simulink model "MSBR_Plant"  (R2021b)
settings: Solver=ode45  StartTime=0.0  StopTime=sim_time  MaxStep=ts_max  RelTol=1e-4
values from neighbouring files (symbols this model uses):
  a_1 = 8.7292e-2/wilson_ratio    (= 0.0087292)    [Whole_Plant_Cool_Pump_Accident_script.m]    (also in Whole_Plant_Fert_Pump_Accident_script.m; Whole_Plant_Fuel_Pump_Accident.m; Whole_Plant_Fuel_Pump_Accident_script.m; Whole_Plant_Reactivity_Accident.m)
  a_2 = 7.3787e-4/wilson_ratio    (= 7.3787e-05)    [Whole_Plant_Cool_Pump_Accident_script.m]    (also in Whole_Plant_Fert_Pump_Accident_script.m; Whole_Plant_Fuel_Pump_Accident.m; Whole_Plant_Fuel_Pump_Accident_script.m; Whole_Plant_Reactivity_Accident.m)
  a_b = 1.656e-5    (= 1.656e-05)    [Whole_Plant_Cool_Pump_Accident_script.m]    (also in Whole_Plant_Fert_Pump_Accident_script.m; Whole_Plant_Fuel_Pump_Accident.m; Whole_Plant_Fuel_Pump_Accident_script.m; Whole_Plant_Reactivity_Accident.m)
  a_f = -8.172e-5    (= -8.172e-05)    [Whole_Plant_Cool_Pump_Accident_script.m]    (also in Whole_Plant_Fert_Pump_Accident_script.m; Whole_Plant_Fuel_Pump_Accident.m; Whole_Plant_Fuel_Pump_Accident_script.m; Whole_Plant_Reactivity_Accident.m)
  a_g = 2.016e-5    (= 2.016e-05)    [Whole_Plant_Cool_Pump_Accident_script.m]    (also in Whole_Plant_Fert_Pump_Accident_script.m; Whole_Plant_Fuel_Pump_Accident.m; Whole_Plant_Fuel_Pump_Accident_script.m; Whole_Plant_Reactivity_Accident.m)
  A_s = pi()*((D_OTSG_i^2)/4) - A_w_OTSG - A_p_OTSG    [Whole_Plant_Cool_Pump_Accident_script.m]    (also in Whole_Plant_Fert_Pump_Accident_script.m; Whole_Plant_Fuel_Pump_Accident.m; Whole_Plant_Fuel_Pump_Accident_script.m; Whole_Plant_Reactivity_Accident.m)
  alpha_co = 316.2    [Whole_Plant_Cool_Pump_Accident_script.m]    (also in Whole_Plant_Fert_Pump_Accident_script.m; Whole_Plant_Fuel_Pump_Accident.m; Whole_Plant_Fuel_Pump_Accident_script.m; Whole_Plant_Reactivity_Accident.m)
  beta = [2.290e-04, 8.320e-04, 7.100e-04, 8.520e-04, 1.710e-04, 1.020e-04]    [Whole_Plant_Cool_Pump_Accident_script.m]    (also in Whole_Plant_Fert_Pump_Accident_script.m; Whole_Plant_Fuel_Pump_Accident.m; Whole_Plant_Fuel_Pump_Accident_script.m; Whole_Plant_Reactivity_Accident.m)
  beta_co = 68.0958    [Whole_Plant_Cool_Pump_Accident_script.m]    (also in Whole_Plant_Fert_Pump_Accident_script.m; Whole_Plant_Fuel_Pump_Accident.m; Whole_Plant_Fuel_Pump_Accident_script.m; Whole_Plant_Reactivity_Accident.m)
  beta_t = sum(beta)    [Whole_Plant_Cool_Pump_Accident_script.m]    (also in Whole_Plant_Fert_Pump_Accident_script.m; Whole_Plant_Fuel_Pump_Accident.m; Whole_Plant_Fuel_Pump_Accident_script.m; Whole_Plant_Reactivity_Accident.m)
  C_nc_X_A_nc = 12.8    [Whole_Plant_Cool_Pump_Accident_script.m]    (also in Whole_Plant_Fert_Pump_Accident_script.m; Whole_Plant_Fuel_Pump_Accident.m; Whole_Plant_Fuel_Pump_Accident_script.m; Whole_Plant_Reactivity_Accident.m)
  C_pcw = 0.0042    [Whole_Plant_Cool_Pump_Accident_script.m]    (also in Whole_Plant_Fert_Pump_Accident_script.m; Whole_Plant_Fuel_Pump_Accident.m; Whole_Plant_Fuel_Pump_Accident_script.m; Whole_Plant_Reactivity_Accident.m)
  C_rh_X_A_rh = 33    [Whole_Plant_Cool_Pump_Accident_script.m]    (also in Whole_Plant_Fert_Pump_Accident_script.m; Whole_Plant_Fuel_Pump_Accident.m; Whole_Plant_Fuel_Pump_Accident_script.m; Whole_Plant_Reactivity_Accident.m)
  C_v = 0.84    [Whole_Plant_Cool_Pump_Accident_script.m]    (also in Whole_Plant_Fert_Pump_Accident_script.m; Whole_Plant_Fuel_Pump_Accident.m; Whole_Plant_Fuel_Pump_Accident_script.m; Whole_Plant_Reactivity_Accident.m)
  ce1 = 1.2471e-07    [Whole_Plant_Cool_Pump_Accident_script.m]    (also in Whole_Plant_Fert_Pump_Accident_script.m; Whole_Plant_Fuel_Pump_Accident.m; Whole_Plant_Fuel_Pump_Accident_script.m; Whole_Plant_Reactivity_Accident.m)
  ce2 = 5.3816e-14    [Whole_Plant_Cool_Pump_Accident_script.m]    (also in Whole_Plant_Fert_Pump_Accident_script.m; Whole_Plant_Fuel_Pump_Accident.m; Whole_Plant_Fuel_Pump_Accident_script.m; Whole_Plant_Reactivity_Accident.m)
  ce3 = 3.3721e-08    [Whole_Plant_Cool_Pump_Accident_script.m]    (also in Whole_Plant_Fert_Pump_Accident_script.m; Whole_Plant_Fuel_Pump_Accident.m; Whole_Plant_Fuel_Pump_Accident_script.m; Whole_Plant_Reactivity_Accident.m)
  Cp_fw = XSteam('Cp_pT',P_set*10,T_fw)/1000    [Whole_Plant_Cool_Pump_Accident_script.m]    (also in Whole_Plant_Fert_Pump_Accident_script.m; Whole_Plant_Fuel_Pump_Accident.m; Whole_Plant_Fuel_Pump_Accident_script.m; Whole_Plant_Reactivity_Accident.m)
  Cp_p = Cp_sec    (= 0.001716588)    [Whole_Plant_Cool_Pump_Accident_script.m]    (also in Whole_Plant_Fert_Pump_Accident_script.m; Whole_Plant_Fuel_Pump_Accident.m; Whole_Plant_Fuel_Pump_Accident_script.m; Whole_Plant_Reactivity_Accident.m)
  Cp_rh = 0.0021520    (= 0.002152)    [Whole_Plant_Cool_Pump_Accident_script.m]    (also in Whole_Plant_Fert_Pump_Accident_script.m; Whole_Plant_Fuel_Pump_Accident.m; Whole_Plant_Fuel_Pump_Accident_script.m; Whole_Plant_Reactivity_Accident.m)
  Cp_s = XSteam('Cp_pT',P_s*10,T_s)/1000    [Whole_Plant_Cool_Pump_Accident_script.m]    (also in Whole_Plant_Fert_Pump_Accident_script.m; Whole_Plant_Fuel_Pump_Accident.m; Whole_Plant_Fuel_Pump_Accident_script.m; Whole_Plant_Reactivity_Accident.m)
  Cp_sc = XSteam('Cp_pT',P_set*10,T_sc2)/1000    [Whole_Plant_Cool_Pump_Accident_script.m]    (also in Whole_Plant_Fert_Pump_Accident_script.m; Whole_Plant_Fuel_Pump_Accident.m; Whole_Plant_Fuel_Pump_Accident_script.m; Whole_Plant_Reactivity_Accident.m)
  Cp_w = 468.992e-6    (= 0.000468992)    [Whole_Plant_Cool_Pump_Accident_script.m]    (also in Whole_Plant_Fert_Pump_Accident_script.m; Whole_Plant_Fuel_Pump_Accident.m; Whole_Plant_Fuel_Pump_Accident_script.m; Whole_Plant_Reactivity_Accident.m)
  D_it = D_ot-2*T_th    (= 0.014147)    [Whole_Plant_Cool_Pump_Accident_script.m]    (also in Whole_Plant_Fert_Pump_Accident_script.m; Whole_Plant_Fuel_Pump_Accident.m; Whole_Plant_Fuel_Pump_Accident_script.m; Whole_Plant_Reactivity_Accident.m)
  D_ot = 0.015875    [Whole_Plant_Cool_Pump_Accident_script.m]    (also in Whole_Plant_Fert_Pump_Accident_script.m; Whole_Plant_Fuel_Pump_Accident.m; Whole_Plant_Fuel_Pump_Accident_script.m; Whole_Plant_Reactivity_Accident.m)
  dHs_dPs = c(1)    [Whole_Plant_Cool_Pump_Accident_script.m]    (also in Whole_Plant_Fert_Pump_Accident_script.m; Whole_Plant_Fuel_Pump_Accident.m; Whole_Plant_Fuel_Pump_Accident_script.m; Whole_Plant_Reactivity_Accident.m)
  eta_hp_isen = 0.861    [Whole_Plant_Cool_Pump_Accident_script.m]    (also in Whole_Plant_Fert_Pump_Accident_script.m; Whole_Plant_Fuel_Pump_Accident.m; Whole_Plant_Fuel_Pump_Accident_script.m; Whole_Plant_Reactivity_Accident.m)
  eta_lp_isen = 0.861    [Whole_Plant_Cool_Pump_Accident_script.m]    (also in Whole_Plant_Fert_Pump_Accident_script.m; Whole_Plant_Fuel_Pump_Accident.m; Whole_Plant_Fuel_Pump_Accident_script.m; Whole_Plant_Reactivity_Accident.m)
  gamma_I = 5.1135e-2    (= 0.051135)    [Whole_Plant_Cool_Pump_Accident_script.m]    (also in Whole_Plant_Fert_Pump_Accident_script.m; Whole_Plant_Fuel_Pump_Accident.m; Whole_Plant_Fuel_Pump_Accident_script.m; Whole_Plant_Reactivity_Accident.m)
  gamma_Xe = 1.1628e-2    (= 0.011628)    [Whole_Plant_Cool_Pump_Accident_script.m]    (also in Whole_Plant_Fert_Pump_Accident_script.m; Whole_Plant_Fuel_Pump_Accident.m; Whole_Plant_Fuel_Pump_Accident_script.m; Whole_Plant_Reactivity_Accident.m)
  H_co0 = 0.149    [Whole_Plant_Cool_Pump_Accident_script.m]    (also in Whole_Plant_Fert_Pump_Accident_script.m; Whole_Plant_Fuel_Pump_Accident.m; Whole_Plant_Fuel_Pump_Accident_script.m; Whole_Plant_Reactivity_Accident.m)
  H_f_co0 = 0.149    [Whole_Plant_Cool_Pump_Accident_script.m]    (also in Whole_Plant_Fert_Pump_Accident_script.m; Whole_Plant_Fuel_Pump_Accident.m; Whole_Plant_Fuel_Pump_Accident_script.m; Whole_Plant_Reactivity_Accident.m)
  H_fg_co0 = 2.35    [Whole_Plant_Cool_Pump_Accident_script.m]    (also in Whole_Plant_Fert_Pump_Accident_script.m; Whole_Plant_Fuel_Pump_Accident.m; Whole_Plant_Fuel_Pump_Accident_script.m; Whole_Plant_Reactivity_Accident.m)
  H_fgrh0 = (XSteam('hV_p', P_s*1e1) - XSteam('hL_p', P_s*1e1))/1e3    [Whole_Plant_Cool_Pump_Accident_script.m]    (also in Whole_Plant_Fert_Pump_Accident_script.m; Whole_Plant_Fuel_Pump_Accident.m; Whole_Plant_Fuel_Pump_Accident_script.m; Whole_Plant_Reactivity_Accident.m)
  H_frh0 = XSteam('hL_p', P_s*1e1)/1e3    [Whole_Plant_Cool_Pump_Accident_script.m]    (also in Whole_Plant_Fert_Pump_Accident_script.m; Whole_Plant_Fuel_Pump_Accident.m; Whole_Plant_Fuel_Pump_Accident_script.m; Whole_Plant_Reactivity_Accident.m)
  h_fwh1 = 0.5927    [Whole_Plant_Cool_Pump_Accident_script.m]    (also in Whole_Plant_Fert_Pump_Accident_script.m; Whole_Plant_Fuel_Pump_Accident.m; Whole_Plant_Fuel_Pump_Accident_script.m; Whole_Plant_Reactivity_Accident.m)
  H_fwh10 = 0.46009    [Whole_Plant_Cool_Pump_Accident_script.m]    (also in Whole_Plant_Fert_Pump_Accident_script.m; Whole_Plant_Fuel_Pump_Accident.m; Whole_Plant_Fuel_Pump_Accident_script.m; Whole_Plant_Reactivity_Accident.m)
  h_fwh2 = 1.230803    [Whole_Plant_Cool_Pump_Accident_script.m]    (also in Whole_Plant_Fert_Pump_Accident_script.m; Whole_Plant_Fuel_Pump_Accident.m; Whole_Plant_Fuel_Pump_Accident_script.m; Whole_Plant_Reactivity_Accident.m)
  H_fwh20 = 0.6784    [Whole_Plant_Cool_Pump_Accident_script.m]    (also in Whole_Plant_Fert_Pump_Accident_script.m; Whole_Plant_Fuel_Pump_Accident.m; Whole_Plant_Fuel_Pump_Accident_script.m; Whole_Plant_Reactivity_Accident.m)
  H_grh0 = 2.8029    [Whole_Plant_Cool_Pump_Accident_script.m]    (also in Whole_Plant_Fert_Pump_Accident_script.m; Whole_Plant_Fuel_Pump_Accident.m; Whole_Plant_Fuel_Pump_Accident_script.m; Whole_Plant_Reactivity_Accident.m)
  H_hp_isen0 = 2.5111    [Whole_Plant_Cool_Pump_Accident_script.m]    (also in Whole_Plant_Fert_Pump_Accident_script.m; Whole_Plant_Fuel_Pump_Accident.m; Whole_Plant_Fuel_Pump_Accident_script.m; Whole_Plant_Reactivity_Accident.m)
  H_hpt_out = 2.6201    [Whole_Plant_Cool_Pump_Accident_script.m]    (also in Whole_Plant_Fert_Pump_Accident_script.m; Whole_Plant_Fuel_Pump_Accident.m; Whole_Plant_Fuel_Pump_Accident_script.m; Whole_Plant_Reactivity_Accident.m)
  H_lp_isen = 958.4*1054.35e-6/0.45359237    (= 2.22774699671)    [Whole_Plant_Cool_Pump_Accident_script.m]    (also in Whole_Plant_Fert_Pump_Accident_script.m; Whole_Plant_Fuel_Pump_Accident.m; Whole_Plant_Fuel_Pump_Accident_script.m; Whole_Plant_Reactivity_Accident.m)
  H_lpt_out = 2.3089    [Whole_Plant_Cool_Pump_Accident_script.m]    (also in Whole_Plant_Fert_Pump_Accident_script.m; Whole_Plant_Fuel_Pump_Accident.m; Whole_Plant_Fuel_Pump_Accident_script.m; Whole_Plant_Reactivity_Accident.m)
  H_nc = XSteam('h_pT', P_s*10, T_s)/1000    [Whole_Plant_Cool_Pump_Accident_script.m]    (also in Whole_Plant_Fert_Pump_Accident_script.m; Whole_Plant_Fuel_Pump_Accident.m; Whole_Plant_Fuel_Pump_Accident_script.m; Whole_Plant_Reactivity_Accident.m)
  h_pw = h_s    (= 0.02555)    [Whole_Plant_Cool_Pump_Accident_script.m]    (also in Whole_Plant_Fert_Pump_Accident_script.m; Whole_Plant_Fuel_Pump_Accident.m; Whole_Plant_Fuel_Pump_Accident_script.m; Whole_Plant_Reactivity_Accident.m)
  H_rh = 2.8115    [Whole_Plant_Cool_Pump_Accident_script.m]    (also in Whole_Plant_Fert_Pump_Accident_script.m; Whole_Plant_Fuel_Pump_Accident.m; Whole_Plant_Fuel_Pump_Accident_script.m; Whole_Plant_Reactivity_Accident.m)
  h_wb = 13349.334646671E-6    (= 0.0133493346467)    [Whole_Plant_Cool_Pump_Accident_script.m]    (also in Whole_Plant_Fert_Pump_Accident_script.m; Whole_Plant_Fuel_Pump_Accident.m; Whole_Plant_Fuel_Pump_Accident_script.m; Whole_Plant_Reactivity_Accident.m)
  h_ws = 5732.378387768E-6    (= 0.00573237838777)    [Whole_Plant_Cool_Pump_Accident_script.m]    (also in Whole_Plant_Fert_Pump_Accident_script.m; Whole_Plant_Fuel_Pump_Accident.m; Whole_Plant_Fuel_Pump_Accident_script.m; Whole_Plant_Reactivity_Accident.m)
  h_wsc = 8385.005556375E-6    (= 0.00838500555638)    [Whole_Plant_Cool_Pump_Accident_script.m]    (also in Whole_Plant_Fert_Pump_Accident_script.m; Whole_Plant_Fuel_Pump_Accident.m; Whole_Plant_Fuel_Pump_Accident_script.m; Whole_Plant_Reactivity_Accident.m)
  hA_bg = A_fert*h_bg    (= 2.76411813627)    [Whole_Plant_Cool_Pump_Accident_script.m]    (also in Whole_Plant_Fert_Pump_Accident_script.m; Whole_Plant_Fuel_Pump_Accident.m; Whole_Plant_Fuel_Pump_Accident_script.m; Whole_Plant_Reactivity_Accident.m)
  hA_co0 = 140    [Whole_Plant_Cool_Pump_Accident_script.m]    (also in Whole_Plant_Fert_Pump_Accident_script.m; Whole_Plant_Fuel_Pump_Accident.m; Whole_Plant_Fuel_Pump_Accident_script.m; Whole_Plant_Reactivity_Accident.m)
  hA_fg_dn = h_fg*A_fuel_down    [Whole_Plant_Cool_Pump_Accident_script.m]    (also in Whole_Plant_Fert_Pump_Accident_script.m; Whole_Plant_Fuel_Pump_Accident.m; Whole_Plant_Fuel_Pump_Accident_script.m; Whole_Plant_Reactivity_Accident.m)
  hA_fg_up = h_fg*A_fuel_up    [Whole_Plant_Cool_Pump_Accident_script.m]    (also in Whole_Plant_Fert_Pump_Accident_script.m; Whole_Plant_Fuel_Pump_Accident.m; Whole_Plant_Fuel_Pump_Accident_script.m; Whole_Plant_Reactivity_Accident.m)
  hA_p_bhx1 = [h_pb*A_pbhx/2,h_pb*A_pbhx/2]    [Whole_Plant_Cool_Pump_Accident_script.m]    (also in Whole_Plant_Fert_Pump_Accident_script.m; Whole_Plant_Fuel_Pump_Accident.m; Whole_Plant_Fuel_Pump_Accident_script.m; Whole_Plant_Reactivity_Accident.m)
  hA_p_bhx2 = hA_p_bhx1    [Whole_Plant_Cool_Pump_Accident_script.m]    (also in Whole_Plant_Fert_Pump_Accident_script.m; Whole_Plant_Fuel_Pump_Accident.m; Whole_Plant_Fuel_Pump_Accident_script.m; Whole_Plant_Reactivity_Accident.m)
  hA_p_bhx3 = hA_p_bhx1    [Whole_Plant_Cool_Pump_Accident_script.m]    (also in Whole_Plant_Fert_Pump_Accident_script.m; Whole_Plant_Fuel_Pump_Accident.m; Whole_Plant_Fuel_Pump_Accident_script.m; Whole_Plant_Reactivity_Accident.m)
  hA_p_bhx4 = hA_p_bhx1    [Whole_Plant_Cool_Pump_Accident_script.m]    (also in Whole_Plant_Fert_Pump_Accident_script.m; Whole_Plant_Fuel_Pump_Accident.m; Whole_Plant_Fuel_Pump_Accident_script.m; Whole_Plant_Reactivity_Accident.m)
  hA_p_fhx1 = [h_p*A_pfhx_dn/2,h_p*A_pfhx_dn/2,h_p*A_pfhx_up/2,h_p*A_pfhx_up/2]    [Whole_Plant_Cool_Pump_Accident_script.m]    (also in Whole_Plant_Fert_Pump_Accident_script.m; Whole_Plant_Fuel_Pump_Accident.m; Whole_Plant_Fuel_Pump_Accident_script.m; Whole_Plant_Reactivity_Accident.m)
  hA_p_fhx2 = hA_p_fhx1    [Whole_Plant_Cool_Pump_Accident_script.m]    (also in Whole_Plant_Fert_Pump_Accident_script.m; Whole_Plant_Fuel_Pump_Accident.m; Whole_Plant_Fuel_Pump_Accident_script.m; Whole_Plant_Reactivity_Accident.m)
  hA_p_fhx3 = hA_p_fhx1    [Whole_Plant_Cool_Pump_Accident_script.m]    (also in Whole_Plant_Fert_Pump_Accident_script.m; Whole_Plant_Fuel_Pump_Accident.m; Whole_Plant_Fuel_Pump_Accident_script.m; Whole_Plant_Reactivity_Accident.m)
  hA_p_fhx4 = hA_p_fhx1    [Whole_Plant_Cool_Pump_Accident_script.m]    (also in Whole_Plant_Fert_Pump_Accident_script.m; Whole_Plant_Fuel_Pump_Accident.m; Whole_Plant_Fuel_Pump_Accident_script.m; Whole_Plant_Reactivity_Accident.m)
  hA_s_bhx1 = [h_sb*A_sbhx/2,h_sb*A_sbhx/2]    [Whole_Plant_Cool_Pump_Accident_script.m]    (also in Whole_Plant_Fert_Pump_Accident_script.m; Whole_Plant_Fuel_Pump_Accident.m; Whole_Plant_Fuel_Pump_Accident_script.m; Whole_Plant_Reactivity_Accident.m)
  hA_s_bhx2 = hA_s_bhx1    [Whole_Plant_Cool_Pump_Accident_script.m]    (also in Whole_Plant_Fert_Pump_Accident_script.m; Whole_Plant_Fuel_Pump_Accident.m; Whole_Plant_Fuel_Pump_Accident_script.m; Whole_Plant_Reactivity_Accident.m)
  hA_s_bhx3 = hA_s_bhx1    [Whole_Plant_Cool_Pump_Accident_script.m]    (also in Whole_Plant_Fert_Pump_Accident_script.m; Whole_Plant_Fuel_Pump_Accident.m; Whole_Plant_Fuel_Pump_Accident_script.m; Whole_Plant_Reactivity_Accident.m)
  hA_s_bhx4 = hA_s_bhx1    [Whole_Plant_Cool_Pump_Accident_script.m]    (also in Whole_Plant_Fert_Pump_Accident_script.m; Whole_Plant_Fuel_Pump_Accident.m; Whole_Plant_Fuel_Pump_Accident_script.m; Whole_Plant_Reactivity_Accident.m)
  hA_s_fhx1 = [h_s*A_sfhx_up/2,h_s*A_sfhx_up/2,h_s*A_sfhx_dn/2,h_s*A_sfhx_dn/2]    [Whole_Plant_Cool_Pump_Accident_script.m]    (also in Whole_Plant_Fert_Pump_Accident_script.m; Whole_Plant_Fuel_Pump_Accident.m; Whole_Plant_Fuel_Pump_Accident_script.m; Whole_Plant_Reactivity_Accident.m)
  hA_s_fhx2 = hA_s_fhx1    [Whole_Plant_Cool_Pump_Accident_script.m]    (also in Whole_Plant_Fert_Pump_Accident_script.m; Whole_Plant_Fuel_Pump_Accident.m; Whole_Plant_Fuel_Pump_Accident_script.m; Whole_Plant_Reactivity_Accident.m)
  hA_s_fhx3 = hA_s_fhx1    [Whole_Plant_Cool_Pump_Accident_script.m]    (also in Whole_Plant_Fert_Pump_Accident_script.m; Whole_Plant_Fuel_Pump_Accident.m; Whole_Plant_Fuel_Pump_Accident_script.m; Whole_Plant_Reactivity_Accident.m)
  hA_s_fhx4 = hA_s_fhx1    [Whole_Plant_Cool_Pump_Accident_script.m]    (also in Whole_Plant_Fert_Pump_Accident_script.m; Whole_Plant_Fuel_Pump_Accident.m; Whole_Plant_Fuel_Pump_Accident_script.m; Whole_Plant_Reactivity_Accident.m)
  I_0 = gamma_I*Sigma_f_msbr*phi_0/lam_I    (= 1.30000734126e+17)    [Whole_Plant_Cool_Pump_Accident_script.m]    (also in Whole_Plant_Fert_Pump_Accident_script.m; Whole_Plant_Fuel_Pump_Accident.m; Whole_Plant_Fuel_Pump_Accident_script.m; Whole_Plant_Reactivity_Accident.m)
  k_1 = 0.5    [Whole_Plant_Cool_Pump_Accident_script.m]    (also in Whole_Plant_Fert_Pump_Accident_script.m; Whole_Plant_Fuel_Pump_Accident.m; Whole_Plant_Fuel_Pump_Accident_script.m; Whole_Plant_Reactivity_Accident.m)
  K_1 = e(1)    [Whole_Plant_Cool_Pump_Accident_script.m]    (also in Whole_Plant_Fert_Pump_Accident_script.m; Whole_Plant_Fuel_Pump_Accident.m; Whole_Plant_Fuel_Pump_Accident_script.m; Whole_Plant_Reactivity_Accident.m)
  k_1b = 0.5    [Whole_Plant_Cool_Pump_Accident_script.m]    (also in Whole_Plant_Fert_Pump_Accident_script.m; Whole_Plant_Fuel_Pump_Accident.m; Whole_Plant_Fuel_Pump_Accident_script.m; Whole_Plant_Reactivity_Accident.m)
  k_2 = 0.5    [Whole_Plant_Cool_Pump_Accident_script.m]    (also in Whole_Plant_Fert_Pump_Accident_script.m; Whole_Plant_Fuel_Pump_Accident.m; Whole_Plant_Fuel_Pump_Accident_script.m; Whole_Plant_Reactivity_Accident.m)
  k_2b = 0.5    [Whole_Plant_Cool_Pump_Accident_script.m]    (also in Whole_Plant_Fert_Pump_Accident_script.m; Whole_Plant_Fuel_Pump_Accident.m; Whole_Plant_Fuel_Pump_Accident_script.m; Whole_Plant_Reactivity_Accident.m)
  k_3 = 0.5    [Whole_Plant_Cool_Pump_Accident_script.m]    (also in Whole_Plant_Fert_Pump_Accident_script.m; Whole_Plant_Fuel_Pump_Accident.m; Whole_Plant_Fuel_Pump_Accident_script.m; Whole_Plant_Reactivity_Accident.m)
  k_4 = 0.5    [Whole_Plant_Cool_Pump_Accident_script.m]    (also in Whole_Plant_Fert_Pump_Accident_script.m; Whole_Plant_Fuel_Pump_Accident.m; Whole_Plant_Fuel_Pump_Accident_script.m; Whole_Plant_Reactivity_Accident.m)
  K_4 = b(1)    [Whole_Plant_Cool_Pump_Accident_script.m]    (also in Whole_Plant_Fert_Pump_Accident_script.m; Whole_Plant_Fuel_Pump_Accident.m; Whole_Plant_Fuel_Pump_Accident_script.m; Whole_Plant_Reactivity_Accident.m)
  K_5 = a(1)    [Whole_Plant_Cool_Pump_Accident_script.m]    (also in Whole_Plant_Fert_Pump_Accident_script.m; Whole_Plant_Fuel_Pump_Accident.m; Whole_Plant_Fuel_Pump_Accident_script.m; Whole_Plant_Reactivity_Accident.m)
  K_b = d(1)    [Whole_Plant_Cool_Pump_Accident_script.m]    (also in Whole_Plant_Fert_Pump_Accident_script.m; Whole_Plant_Fuel_Pump_Accident.m; Whole_Plant_Fuel_Pump_Accident_script.m; Whole_Plant_Reactivity_Accident.m)
  k_b1 = (K_B/2)/K    (= 0.0089463103122)    [Whole_Plant_Cool_Pump_Accident_script.m]    (also in Whole_Plant_Fert_Pump_Accident_script.m; Whole_Plant_Fuel_Pump_Accident.m; Whole_Plant_Fuel_Pump_Accident_script.m; Whole_Plant_Reactivity_Accident.m)
  k_b2 = k_b1    (= 0.0089463103122)    [Whole_Plant_Cool_Pump_Accident_script.m]    (also in Whole_Plant_Fert_Pump_Accident_script.m; Whole_Plant_Fuel_Pump_Accident.m; Whole_Plant_Fuel_Pump_Accident_script.m; Whole_Plant_Reactivity_Accident.m)
  K_bhp = 0.1634    [Whole_Plant_Cool_Pump_Accident_script.m]    (also in Whole_Plant_Fert_Pump_Accident_script.m; Whole_Plant_Fuel_Pump_Accident.m; Whole_Plant_Fuel_Pump_Accident_script.m; Whole_Plant_Reactivity_Accident.m)
  K_blp = 0.2174    [Whole_Plant_Cool_Pump_Accident_script.m]    (also in Whole_Plant_Fert_Pump_Accident_script.m; Whole_Plant_Fuel_Pump_Accident.m; Whole_Plant_Fuel_Pump_Accident_script.m; Whole_Plant_Reactivity_Accident.m)
  k_f1 = ((1 - K_G - K_B - K_Ba)/4)/K    (= 0.226055463576)    [Whole_Plant_Cool_Pump_Accident_script.m]    (also in Whole_Plant_Fert_Pump_Accident_script.m; Whole_Plant_Fuel_Pump_Accident.m; Whole_Plant_Fuel_Pump_Accident_script.m; Whole_Plant_Reactivity_Accident.m)
  k_f2 = k_f1    (= 0.226055463576)    [Whole_Plant_Cool_Pump_Accident_script.m]    (also in Whole_Plant_Fert_Pump_Accident_script.m; Whole_Plant_Fuel_Pump_Accident.m; Whole_Plant_Fuel_Pump_Accident_script.m; Whole_Plant_Reactivity_Accident.m)
  k_f3 = k_f1    (= 0.226055463576)    [Whole_Plant_Cool_Pump_Accident_script.m]    (also in Whole_Plant_Fert_Pump_Accident_script.m; Whole_Plant_Fuel_Pump_Accident.m; Whole_Plant_Fuel_Pump_Accident_script.m; Whole_Plant_Reactivity_Accident.m)
  k_f4 = k_f1    (= 0.226055463576)    [Whole_Plant_Cool_Pump_Accident_script.m]    (also in Whole_Plant_Fert_Pump_Accident_script.m; Whole_Plant_Fuel_Pump_Accident.m; Whole_Plant_Fuel_Pump_Accident_script.m; Whole_Plant_Reactivity_Accident.m)
  k_g1 = ((K_G*K_fuel)/2)/K    (= 0.0346590586566)    [Whole_Plant_Cool_Pump_Accident_script.m]    (also in Whole_Plant_Fert_Pump_Accident_script.m; Whole_Plant_Fuel_Pump_Accident.m; Whole_Plant_Fuel_Pump_Accident_script.m; Whole_Plant_Reactivity_Accident.m)
  k_g2 = k_g1    (= 0.0346590586566)    [Whole_Plant_Cool_Pump_Accident_script.m]    (also in Whole_Plant_Fert_Pump_Accident_script.m; Whole_Plant_Fuel_Pump_Accident.m; Whole_Plant_Fuel_Pump_Accident_script.m; Whole_Plant_Reactivity_Accident.m)
  k_g3 = (K_G*(1-K_fuel))/K    (= 0.00856740775781)    [Whole_Plant_Cool_Pump_Accident_script.m]    (also in Whole_Plant_Fert_Pump_Accident_script.m; Whole_Plant_Fuel_Pump_Accident.m; Whole_Plant_Fuel_Pump_Accident_script.m; Whole_Plant_Reactivity_Accident.m)
  K_sc = f(1)    [Whole_Plant_Cool_Pump_Accident_script.m]    (also in Whole_Plant_Fert_Pump_Accident_script.m; Whole_Plant_Fuel_Pump_Accident.m; Whole_Plant_Fuel_Pump_Accident_script.m; Whole_Plant_Reactivity_Accident.m)
  L = 22.0    (= 22)    [Whole_Plant_Cool_Pump_Accident_script.m]    (also in Whole_Plant_Fert_Pump_Accident_script.m; Whole_Plant_Fuel_Pump_Accident.m; Whole_Plant_Fuel_Pump_Accident_script.m; Whole_Plant_Reactivity_Accident.m)
  L_b = 1.9    [Whole_Plant_Cool_Pump_Accident_script.m]    (also in Whole_Plant_Fert_Pump_Accident_script.m; Whole_Plant_Fuel_Pump_Accident.m; Whole_Plant_Fuel_Pump_Accident_script.m; Whole_Plant_Reactivity_Accident.m)
  L_s = 16.53    [Whole_Plant_Cool_Pump_Accident_script.m]    (also in Whole_Plant_Fert_Pump_Accident_script.m; Whole_Plant_Fuel_Pump_Accident.m; Whole_Plant_Fuel_Pump_Accident_script.m; Whole_Plant_Reactivity_Accident.m)
  L_sc = L-L_b-L_s    (= 3.57)    [Whole_Plant_Cool_Pump_Accident_script.m]    (also in Whole_Plant_Fert_Pump_Accident_script.m; Whole_Plant_Fuel_Pump_Accident.m; Whole_Plant_Fuel_Pump_Accident_script.m; Whole_Plant_Reactivity_Accident.m)
  Lam = 3.3e-4    (= 0.00033)    [Whole_Plant_Cool_Pump_Accident_script.m]    (also in Whole_Plant_Fert_Pump_Accident_script.m; Whole_Plant_Fuel_Pump_Accident.m; Whole_Plant_Fuel_Pump_Accident_script.m; Whole_Plant_Reactivity_Accident.m)
  lam = [1.260e-02, 3.370e-02, 1.390e-01, 3.250e-01, 1.130e+00, 2.500e+00]    [Whole_Plant_Cool_Pump_Accident_script.m]    (also in Whole_Plant_Fert_Pump_Accident_script.m; Whole_Plant_Fuel_Pump_Accident.m; Whole_Plant_Fuel_Pump_Accident_script.m; Whole_Plant_Reactivity_Accident.m)
  lam_bubl = 2.0e-2    (= 0.02)    [Whole_Plant_Cool_Pump_Accident_script.m]    (also in Whole_Plant_Fert_Pump_Accident_script.m; Whole_Plant_Fuel_Pump_Accident.m; Whole_Plant_Fuel_Pump_Accident_script.m; Whole_Plant_Reactivity_Accident.m)
  lam_I = 2.875e-5    (= 2.875e-05)    [Whole_Plant_Cool_Pump_Accident_script.m]    (also in Whole_Plant_Fert_Pump_Accident_script.m; Whole_Plant_Fuel_Pump_Accident.m; Whole_Plant_Fuel_Pump_Accident_script.m; Whole_Plant_Reactivity_Accident.m)
  lam_Xe = 2.0916e-5    (= 2.0916e-05)    [Whole_Plant_Cool_Pump_Accident_script.m]    (also in Whole_Plant_Fert_Pump_Accident_script.m; Whole_Plant_Fuel_Pump_Accident.m; Whole_Plant_Fuel_Pump_Accident_script.m; Whole_Plant_Reactivity_Accident.m)
  m_bm = (W_b1+W_b2+W_b3+W_b4)*time_mixb    (= 2167.1636)    [Whole_Plant_Cool_Pump_Accident_script.m]    (also in Whole_Plant_Fert_Pump_Accident_script.m; Whole_Plant_Fuel_Pump_Accident.m; Whole_Plant_Fuel_Pump_Accident_script.m; Whole_Plant_Reactivity_Accident.m)
  M_cw = 65000    [Whole_Plant_Cool_Pump_Accident_script.m]    (also in Whole_Plant_Fert_Pump_Accident_script.m; Whole_Plant_Fuel_Pump_Accident.m; Whole_Plant_Fuel_Pump_Accident_script.m; Whole_Plant_Reactivity_Accident.m)
  m_fm = (W_f1+W_f2+W_f3+W_f4)*time_mixf    (= 5443.108)    [Whole_Plant_Cool_Pump_Accident_script.m]    (also in Whole_Plant_Fert_Pump_Accident_script.m; Whole_Plant_Fuel_Pump_Accident.m; Whole_Plant_Fuel_Pump_Accident_script.m; Whole_Plant_Reactivity_Accident.m)
  M_hw0 = 10000    [Whole_Plant_Cool_Pump_Accident_script.m]    (also in Whole_Plant_Fert_Pump_Accident_script.m; Whole_Plant_Fuel_Pump_Accident.m; Whole_Plant_Fuel_Pump_Accident_script.m; Whole_Plant_Reactivity_Accident.m)
  m_sm = (W_s1+W_s2+W_s3+W_s4)*time_mixs    (= 8467.056)    [Whole_Plant_Cool_Pump_Accident_script.m]    (also in Whole_Plant_Fert_Pump_Accident_script.m; Whole_Plant_Fuel_Pump_Accident.m; Whole_Plant_Fuel_Pump_Accident_script.m; Whole_Plant_Reactivity_Accident.m)
  M_stm = 0.018    [Whole_Plant_Cool_Pump_Accident_script.m]    (also in Whole_Plant_Fert_Pump_Accident_script.m; Whole_Plant_Fuel_Pump_Accident.m; Whole_Plant_Fuel_Pump_Accident_script.m; Whole_Plant_Reactivity_Accident.m)
  mcp_b1 = mass_bn*Cp_b    (= 4.17494922705)    [Whole_Plant_Cool_Pump_Accident_script.m]    (also in Whole_Plant_Fert_Pump_Accident_script.m; Whole_Plant_Fuel_Pump_Accident.m; Whole_Plant_Fuel_Pump_Accident_script.m; Whole_Plant_Reactivity_Accident.m)
  mcp_b2 = mcp_b1    (= 4.17494922705)    [Whole_Plant_Cool_Pump_Accident_script.m]    (also in Whole_Plant_Fert_Pump_Accident_script.m; Whole_Plant_Fuel_Pump_Accident.m; Whole_Plant_Fuel_Pump_Accident_script.m; Whole_Plant_Reactivity_Accident.m)
  mcp_f1 = mass_fn*Cp_f    (= 5.5019469141)    [Whole_Plant_Cool_Pump_Accident_script.m]    (also in Whole_Plant_Fert_Pump_Accident_script.m; Whole_Plant_Fuel_Pump_Accident.m; Whole_Plant_Fuel_Pump_Accident_script.m; Whole_Plant_Reactivity_Accident.m)
  mcp_f2 = mass_fn*Cp_f    (= 5.5019469141)    [Whole_Plant_Cool_Pump_Accident_script.m]    (also in Whole_Plant_Fert_Pump_Accident_script.m; Whole_Plant_Fuel_Pump_Accident.m; Whole_Plant_Fuel_Pump_Accident_script.m; Whole_Plant_Reactivity_Accident.m)
  mcp_f3 = mass_fn*Cp_f    (= 5.5019469141)    [Whole_Plant_Cool_Pump_Accident_script.m]    (also in Whole_Plant_Fert_Pump_Accident_script.m; Whole_Plant_Fuel_Pump_Accident.m; Whole_Plant_Fuel_Pump_Accident_script.m; Whole_Plant_Reactivity_Accident.m)
  mcp_f4 = mass_fn*Cp_f    (= 5.5019469141)    [Whole_Plant_Cool_Pump_Accident_script.m]    (also in Whole_Plant_Fert_Pump_Accident_script.m; Whole_Plant_Fuel_Pump_Accident.m; Whole_Plant_Fuel_Pump_Accident_script.m; Whole_Plant_Reactivity_Accident.m)
  mcp_g1 = (mass_grap*Cp_g)*K_fuel/2    (= 32.9814988203)    [Whole_Plant_Cool_Pump_Accident_script.m]    (also in Whole_Plant_Fert_Pump_Accident_script.m; Whole_Plant_Fuel_Pump_Accident.m; Whole_Plant_Fuel_Pump_Accident_script.m; Whole_Plant_Reactivity_Accident.m)
  mcp_g2 = mcp_g1    (= 32.9814988203)    [Whole_Plant_Cool_Pump_Accident_script.m]    (also in Whole_Plant_Fert_Pump_Accident_script.m; Whole_Plant_Fuel_Pump_Accident.m; Whole_Plant_Fuel_Pump_Accident_script.m; Whole_Plant_Reactivity_Accident.m)
  mcp_g3 = (mass_grap*Cp_g)*(1-K_fuel)    (= 8.15273004546)    [Whole_Plant_Cool_Pump_Accident_script.m]    (also in Whole_Plant_Fert_Pump_Accident_script.m; Whole_Plant_Fuel_Pump_Accident.m; Whole_Plant_Fuel_Pump_Accident_script.m; Whole_Plant_Reactivity_Accident.m)
  mcp_p_bhx1 = mp_bhx1*Cp_b    [Whole_Plant_Cool_Pump_Accident_script.m]    (also in Whole_Plant_Fert_Pump_Accident_script.m; Whole_Plant_Fuel_Pump_Accident.m; Whole_Plant_Fuel_Pump_Accident_script.m; Whole_Plant_Reactivity_Accident.m)
  mcp_p_bhx2 = mp_bhx2*Cp_b    [Whole_Plant_Cool_Pump_Accident_script.m]    (also in Whole_Plant_Fert_Pump_Accident_script.m; Whole_Plant_Fuel_Pump_Accident.m; Whole_Plant_Fuel_Pump_Accident_script.m; Whole_Plant_Reactivity_Accident.m)
  mcp_p_bhx3 = mp_bhx3*Cp_b    [Whole_Plant_Cool_Pump_Accident_script.m]    (also in Whole_Plant_Fert_Pump_Accident_script.m; Whole_Plant_Fuel_Pump_Accident.m; Whole_Plant_Fuel_Pump_Accident_script.m; Whole_Plant_Reactivity_Accident.m)
  ... (+213 more)
undefined symbols (not defined in the file or in its folder): C0, H_con_table, H_convap_table, H_rh_table, H_rh_table1, H_rh_table2, H_rhvap_table, H_s_table, H_table, P_con_table, P_nc_table, P_rh_table, P_rh_table1, pres_table, rho_rh_table, rho_table, SV_nc_table, SVf_nc_table, temp_table
(part 6 of 13)

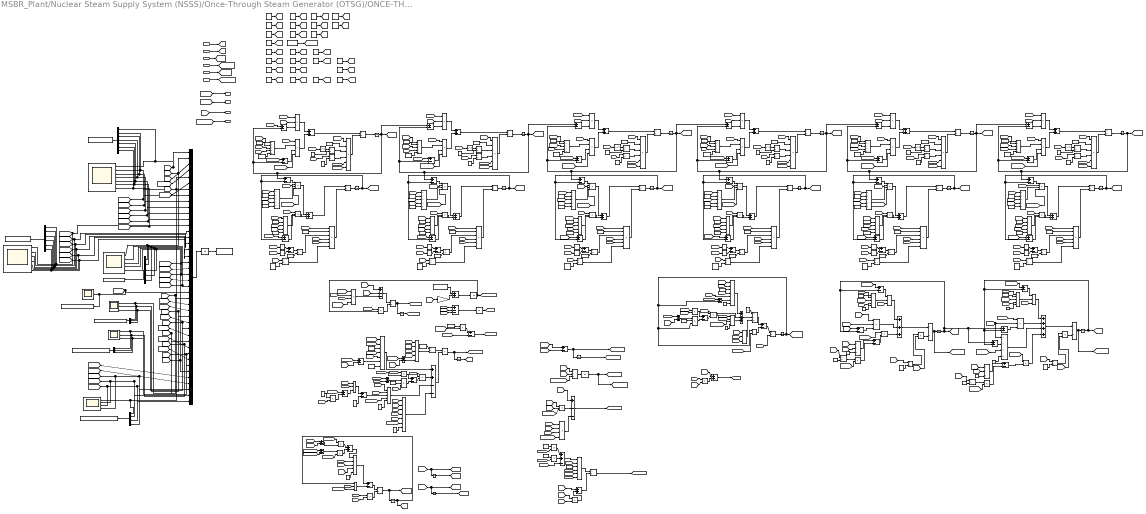
== system MSBR_Plant/Nuclear Steam Supply System (NSSS)/Once-Through Steam Generator (OTSG)/ONCE-THROUGH STEAM GENERATOR ==
  note: Mass and Mass Flow Rate Calculations
  note: Saturated Lump Temperature
  note: Pressure
  note: Water/Steam Level Calculations
  note: OTSG Sub-cooled Lump
  note: OTSG Superheated Steam Lumps
  note: OTSG Wall Lumps
  note: Coolant Salt (Primary) Lumps
  note: Constants
  note: Output
  note: Input
  Coolant Salt Inlet Temp : Inport
  Feedwater Inlet Temp : Inport  Port=2
  Coolant Salt Flow Rate : Inport  Port=3
  Coolant Salt Heat Transfer Frac : Inport  Port=4
  Feedwater Flow Rate : Inport  Port=5
  Pressure Set Point : Inport  Port=6
  Constant : Constant  Value=Cp_p
  Constant1 : Constant  Value=h_pw
  Constant10 : Constant  Value=h_wsc
  Constant{27,29,32,34,37,39,42,44,47,49,52,54,57,59,61,64,66,68,71,73,75,78,80,82,85,87,89,92,94,96,100,105,111,120,127} (35 alike) : Constant  Value=pi
  Constant{28,30,33,35,38,40,43,45,48,50,53,55,58,60,63,65,67,70,72,74,77,79,81,84,86,88,91,93,95,98..99,101..104,106..110,112..113,121..122,124..126} (47 alike) : Constant  Value=2
  Constant11 : Constant  Value=Cp_s
  Constant{114,118..119,128..129} (5 alike) : Constant  Value=0.5
  Constant115 : Constant  Value=25.884875705
  Constant116 : Constant  Value=-1
  Constant117 : Constant
  Constant12 : Constant  Value=A_s
  Constant123 : Constant
  Constant13 : Constant  Value=dHs_dPs
  Constant14 : Constant  Value=Cp_sc
  Constant15 : Constant  Value=rho_sc
  Constant16 : Constant  Value=L
  Constant17 : Constant  Value=K_b
  Constant18 : Constant  Value=K_sc
  Constant19 : Constant  Value=K_1
  Constant2 : Constant  Value=N
  Constant20 : Constant  Value=Z_ss
  Constant21 : Constant  Value=R
  Constant22 : Constant  Value=M_stm
  Constant23 : Constant  Value=K_5
  Constant24 : Constant  Value=X_5
  Constant25 : Constant  Value=K_4
  Constant26 : Constant  Value=X_4
  Constant3 : Constant  Value=D_it
  Constant{31,36,41,46,51,56,62,69,76,83,90,97} (12 alike) : Constant  Value=4
  Constant4 : Constant  Value=rho_p
  Constant5 : Constant  Value=h_ws
  Constant6 : Constant  Value=D_ot
  Constant7 : Constant  Value=Cp_w
  Constant8 : Constant  Value=rho_w
  Constant9 : Constant  Value=h_wb
  Density of Boiling : Scope
  Divide{,7,18,25,32,39,44,52,60,68,76,84,92,94,102,104,115,123,126,131,134} (21 alike) : Product  Inputs=***
  Divide{1,8,19,26,33,40,42,50,58,66,74,82,135} (13 alike) : Product  Inputs=****
  Divide{3,10,14,21,28,35,47,55,63,71,79,87,137} (13 alike) : Product  Inputs=******
  Divide{2,5..6,9,12..13,16..17,20,23..24,27,30..31,34,37..38,41,46,48..49,54,56..57,62,64..65,70,72..73,78,80..81,86,88..91,97,100..101,105,107,117..118,129,136} (47 alike) : Product  Inputs=*/
  Divide{4,11,15,22,29,36,43,45,51,53,59,61,67,69,75,77,83,85,93,103,125} (21 alike) : Product  Inputs=****/
  Divide{96,106,110,133} (4 alike) : Product  Inputs=**/
  Divide{98..99,108..109,113..114,116,120..122,127,130} (12 alike) : Product  Inputs=**
  Divide111 : Product  Inputs=******/
  Divide112 : Product  Inputs=***/
  Divide119 : Product  Inputs=*****
  Divide124 : Product  Inputs=******/
  Divide128 : Product  Inputs=******/
  Divide132 : Product  Inputs=***//
  Divide95 : Product  Inputs=***/
  Feedwater and Steam Flow Rates : Scope  NumInputPorts=4
  Feedwater and Steam Pressures : Scope  NumInputPorts=3
  Feedwater and steam Temps : Scope  NumInputPorts=5
  L_b : Integrator  InitialCondition=L_b
  L_sc : Integrator  InitialCondition=L_sc
  M_shs : Integrator  InitialCondition=A_s*rho_s*L_s
  Minus{,1..12,14..16,18..20,22..24,26..28,30..32,34..35,37..40,42..45,47..48,51,53,55,57..60,63} (48 alike) : Sum  Inputs=+-
  Minus{13,17,21,25,29,33,49,56,61..62,65} (11 alike) : Sum
  Minus36 : Sum  Inputs=++++
  Minus41 : Sum  Inputs=+++
  Minus46 : Sum  Inputs=+++
  Minus50 : Sum  Inputs=+--
  Minus52 : Sum  Inputs=+--
  Minus54 : Sum  Inputs=++--
  Minus64 : Sum  Inputs=+--
  Minus66 : Sum  Inputs=++-
  Multiply : Gain  Gain=12.835
  Mux : Mux  Inputs=42
  Mux1 : Mux  Inputs=7
  Mux2 : Mux  Inputs=6
  Mux3 : Mux  Inputs=5
  Mux4 : Mux  Inputs=3
  Mux5 : Mux  Inputs=3
  Mux6 : Mux
  OTSG Level : Scope  NumInputPorts=3
  OTSG Primary Temps : Scope  NumInputPorts=7
  OTSG Tube Temps : Scope  NumInputPorts=6
  P_s : Integrator  InitialCondition=P_s
  P_sat : Integrator  InitialCondition=P_sat
  P_sc : Integrator  InitialCondition=P_sc
  Plus{,1..6} (7 alike) : Sum
  Product{,1,3..4,6..11} (10 alike) : Product
  Product2 : Product  Inputs=3
  Product5 : Product  Inputs=4
  Square{,1..17} (18 alike) : Math  Operator=square  SaturateOnIntegerOverflow=on
  Sum : Sum  Inputs=+|+
  Sum1 : Sum  Inputs=+|+
  To Workspace : ToWorkspace  VariableName=OTSG_mux  SaveFormat=Timeseries  SampleTime=-1
  To Workspace1 : ToWorkspace  VariableName=OTSG_Primary_Cool_Temps  SaveFormat=Timeseries  SampleTime=-1
  To Workspace2 : ToWorkspace  VariableName=OTSG_Tube_Temps  SaveFormat=Timeseries  SampleTime=-1
  To Workspace3 : ToWorkspace  VariableName=OTSG_Secondary_Temps  SaveFormat=Timeseries  SampleTime=-1
  To Workspace4 : ToWorkspace  VariableName=OTSG_Secondary_Boil_Density  SaveFormat=Timeseries  SampleTime=-1
  To Workspace5 : ToWorkspace  VariableName=OTSG_Secondary_Level  SaveFormat=Timeseries  SampleTime=-1
  To Workspace6 : ToWorkspace  VariableName=OTSG_Secondary_Pressures  SaveFormat=Timeseries  SampleTime=-1
  To Workspace7 : ToWorkspace  VariableName=OTSG_Secondary_Flow_Rates  SaveFormat=Timeseries  SampleTime=-1
  Tp1_otsg : Integrator  InitialCondition=T_p1
  Tp2_otsg : Integrator  InitialCondition=T_p2
  Tp3_otsg : Integrator  InitialCondition=T_p3
  Tp4_otsg : Integrator  InitialCondition=T_p4
  Tp5_otsg : Integrator  InitialCondition=T_p5
  Tp6_otsg : Integrator  InitialCondition=T_p6
  Ts1_otsg : Integrator  InitialCondition=T_s1
  Ts2_otsg : Integrator  InitialCondition=T_s2
  Tsc2_otsg : Integrator  InitialCondition=T_sc2
  Tw1_otsg : Integrator  InitialCondition=T_w1
  Tw2_otsg : Integrator  InitialCondition=T_w2
  Tw3_otsg : Integrator  InitialCondition=T_w3
  Tw4_otsg : Integrator  InitialCondition=T_w4
  Tw5_otsg : Integrator  InitialCondition=T_w5
  Tw6_otsg : Integrator  InitialCondition=T_w6
  Unit Delay : UnitDelay  InitialCondition=rho_b  SampleTime=-1  HasFrameUpgradeWarning=on
  Unit Delay1 : UnitDelay  InitialCondition=L_s  SampleTime=-1  HasFrameUpgradeWarning=on
  Unit Delay2 : UnitDelay  InitialCondition=W_fw  SampleTime=-1  HasFrameUpgradeWarning=on
  Unit Delay3 : UnitDelay  SampleTime=-1  HasFrameUpgradeWarning=on
  Steam Temperature : Outport  VectorParamsAs1DForOutWhenUnconnected=off
  Coolant Salt Outlet Temperature : Outport  Port=2  VectorParamsAs1DForOutWhenUnconnected=off
  Steam Pressure : Outport  Port=3  VectorParamsAs1DForOutWhenUnconnected=off
  Steam Flow Rate : Outport  Port=4  VectorParamsAs1DForOutWhenUnconnected=off
  wires:
  Feedwater Inlet Temp/1 -> [Tfw_in]
  Coolant Salt Inlet Temp/1 -> [Tp_in]
  Coolant Salt Flow Rate/1 -> [Wp_in]
  Coolant Salt Heat Transfer Frac/1 -> [cool_hA_frac]
  Feedwater Flow Rate/1 -> [Wfw_in]
  Pressure Set Point/1 -> [P_set_point]
  Tw1_otsg/1 -> [Tw1_otsg], Minus14/2, Minus12/2
  Ts1_otsg/1 -> [Ts1_otsg], Minus39/2, Minus38/2, Minus37/2
  L_sc/1 -> [L_sc]
  L_b/1 -> [L_b]
  P_sat/1 -> [P_sat]  "Sat Pressure"
  Tsc2_otsg/1 -> Minus47/2, Divide115/3, Product3/1, [Tsc2_otsg]
  Unit Delay/1 -> Product4/2, [rho_b_Ps]
  M_shs/1 -> [M_shs]  "Superheated Steam Mass"
  Unit Delay1/1 -> [L_s]
  Constant/1 -> [Cp_p]
  Constant1/1 -> [h_pw]
  Constant2/1 -> [N]
  Constant3/1 -> [D_it]
  Constant4/1 -> [rho_p]
  Constant5/1 -> [h_ws]
  Constant6/1 -> [D_ot]
  Constant8/1 -> [rho_w]
  Constant7/1 -> [Cp_w]
  Constant9/1 -> [h_wb]
  Constant10/1 -> [h_wsc]
  Constant12/1 -> [A_s]
  Constant11/1 -> [Cp_s]
  Constant13/1 -> [dHs_dPs]
  Constant14/1 -> [Cp_sc]
  Constant15/1 -> [rho_sc]
  Constant16/1 -> [L]
  Constant17/1 -> [K_b]
  Constant18/1 -> [K_sc]
  Constant19/1 -> [K_1]
  Constant20/1 -> [Z_ss]
  Constant21/1 -> [R]
  Constant22/1 -> [M_stm]
  Constant23/1 -> [K_5]
  Constant24/1 -> [X_5]
  Constant25/1 -> [K_4]
  Constant26/1 -> [X_4]
  [Wp_in] -> Divide/1
  [Cp_p] -> Divide/2
  [Tp_in] -> Minus/1
  Minus/1 -> Divide/3
  Divide/1 -> Plus/1
  Divide1/1 -> Plus/2
  [h_pw] -> Divide1/1
  [N] -> Divide4/1
  Constant27/1 -> Divide4/2
  [D_it] -> Divide4/3
  Constant28/1 -> Divide4/5
  Minus1/1 -> Divide1/3
  Plus/1 -> Divide2/1
  Divide3/1 -> Divide2/2
  [N] -> Divide3/1
  Constant29/1 -> Divide3/2
  [D_it] -> Square/1
  Square/1 -> Divide5/1
  [rho_p] -> Divide3/5
  [Cp_p] -> Divide3/6
  Constant31/1 -> Divide5/2
  Constant30/1 -> Divide6/2
  Divide2/1 -> Tp1_otsg/1
  Divide4/1 -> Divide1/2
  Divide5/1 -> Divide3/3
  Divide6/1 -> Divide3/4
  Divide13/1 -> Divide10/4
  Divide12/1 -> Divide10/3
  Divide11/1 -> Divide8/2
  Divide9/1 -> Tp2_otsg/1
  Constant35/1 -> Divide13/2
  Constant36/1 -> Divide12/2
  [Cp_p] -> Divide10/6
  [rho_p] -> Divide10/5
  Square1/1 -> Divide12/1
  [D_it] -> Square1/1
  Constant34/1 -> Divide10/2
  [N] -> Divide10/1
  Divide10/1 -> Divide9/2
  Plus1/1 -> Divide9/1
  Minus3/1 -> Divide8/3
  Constant33/1 -> Divide11/5
  [D_it] -> Divide11/3
  Constant32/1 -> Divide11/2
  [N] -> Divide11/1
  [h_pw] -> Divide8/1
  Divide8/1 -> Plus1/2
  Divide7/1 -> Plus1/1
  Minus2/1 -> Divide7/3
  Tp1_otsg/1 -> Minus2/1, [Tp1_otsg], Minus12/1, Minus1/2, Minus/2
  [Cp_p] -> Divide7/2
  [Wp_in] -> Divide7/1
  [Wp_in] -> Divide18/1
  [Cp_p] -> Divide18/2
  Minus4/1 -> Divide18/3
  Divide18/1 -> Plus2/1
  Divide19/1 -> Plus2/2
  [h_pw] -> Divide19/1
  [N] -> Divide15/1
  Constant37/1 -> Divide15/2
  [D_it] -> Divide15/3
  Constant38/1 -> Divide15/5
  Minus5/1 -> Divide19/3
  Plus2/1 -> Divide20/1
  Divide14/1 -> Divide20/2
  [N] -> Divide14/1
  Constant39/1 -> Divide14/2
  [D_it] -> Square2/1
  Square2/1 -> Divide16/1
  [rho_p] -> Divide14/5
  [Cp_p] -> Divide14/6
  Constant41/1 -> Divide16/2
  Constant40/1 -> Divide17/2
  Divide20/1 -> Tp3_otsg/1
  Divide15/1 -> Divide19/2
  Divide16/1 -> Divide14/3
  Divide17/1 -> Divide14/4
  Divide24/1 -> Divide21/4
  Divide23/1 -> Divide21/3
  Divide22/1 -> Divide26/2
  Divide27/1 -> Tp4_otsg/1
  Constant45/1 -> Divide24/2
  Constant46/1 -> Divide23/2
  [Cp_p] -> Divide21/6
  [rho_p] -> Divide21/5
  Square3/1 -> Divide23/1
  [D_it] -> Square3/1
  Constant44/1 -> Divide21/2
  [N] -> Divide21/1
  Divide21/1 -> Divide27/2
  Plus3/1 -> Divide27/1
  Minus7/1 -> Divide26/3
  Constant43/1 -> Divide22/5
  [D_it] -> Divide22/3
  Constant42/1 -> Divide22/2
  [N] -> Divide22/1
  [h_pw] -> Divide26/1
  Divide26/1 -> Plus3/2
  Divide25/1 -> Plus3/1
  Minus6/1 -> Divide25/3
  [Cp_p] -> Divide25/2
  [Wp_in] -> Divide25/1
  [Wp_in] -> Divide32/1
  [Cp_p] -> Divide32/2
  Minus8/1 -> Divide32/3
  Divide32/1 -> Plus4/1
  Divide33/1 -> Plus4/2
  [h_pw] -> Divide33/1
  [N] -> Divide29/1
  Constant47/1 -> Divide29/2
  [D_it] -> Divide29/3
  Constant48/1 -> Divide29/5
  Minus9/1 -> Divide33/3
  Plus4/1 -> Divide34/1
  Divide28/1 -> Divide34/2
  [N] -> Divide28/1
  Constant49/1 -> Divide28/2
  [D_it] -> Square4/1
  Square4/1 -> Divide30/1
  [rho_p] -> Divide28/5
  [Cp_p] -> Divide28/6
  Constant51/1 -> Divide30/2
  Constant50/1 -> Divide31/2
  Divide34/1 -> Tp5_otsg/1
  Divide29/1 -> Divide33/2
  Divide30/1 -> Divide28/3
  Divide31/1 -> Divide28/4
  Divide38/1 -> Divide35/4
  Divide37/1 -> Divide35/3
  Divide36/1 -> Divide40/2
  Divide41/1 -> Tp6_otsg/1
  Constant55/1 -> Divide38/2
  Constant56/1 -> Divide37/2
  [Cp_p] -> Divide35/6
  [rho_p] -> Divide35/5
  Square5/1 -> Divide37/1
  [D_it] -> Square5/1
  Constant54/1 -> Divide35/2
  [N] -> Divide35/1
  Divide35/1 -> Divide41/2
  Plus5/1 -> Divide41/1
  Minus11/1 -> Divide40/3
  Constant53/1 -> Divide36/5
  [D_it] -> Divide36/3
  Constant52/1 -> Divide36/2
  [N] -> Divide36/1
  [h_pw] -> Divide40/1
  Divide40/1 -> Plus5/2
  Divide39/1 -> Plus5/1
  Minus10/1 -> Divide39/3
  [Cp_p] -> Divide39/2
  [Wp_in] -> Divide39/1
  Constant58/1 -> Divide43/5
  [D_it] -> Divide43/3
  Constant57/1 -> Divide43/2
  [N] -> Divide43/1
  Divide43/1 -> Divide42/3
  [h_pw] -> Divide42/2
  Minus12/1 -> Divide42/1
  Divide42/1 -> Minus13/1
  Divide44/1 -> Minus13/2
  [h_ws] -> Divide44/1
  Divide45/1 -> Divide44/2
  [N] -> Divide45/1
  Constant59/1 -> Divide45/2
  [D_ot] -> Divide45/3
  Constant60/1 -> Divide45/5
  Minus14/1 -> Divide44/3
  Minus13/1 -> Divide46/1
  [D_ot] -> Square6/1
  [D_it] -> Square7/1
  Square6/1 -> Minus15/1
  Square7/1 -> Minus15/2
  Constant62/1 -> Divide48/2
  Minus15/1 -> Divide48/1
  [N] -> Divide47/1
  Constant61/1 -> Divide47/2
  Divide47/1 -> Divide46/2
  Divide48/1 -> Divide47/3
  [rho_w] -> Divide47/4
  [Cp_w] -> Divide47/5
  Divide49/1 -> Divide47/6
  Divide46/1 -> Tw1_otsg/1
  Constant63/1 -> Divide49/2
  Constant70/1 -> Divide57/2
  Divide54/1 -> Tw2_otsg/1
  Divide57/1 -> Divide55/6
  [Cp_w] -> Divide55/5
  [rho_w] -> Divide55/4
  Divide56/1 -> Divide55/3
  Divide55/1 -> Divide54/2
  Constant68/1 -> Divide55/2
  [N] -> Divide55/1
  Minus19/1 -> Divide56/1
  Constant69/1 -> Divide56/2
  Square9/1 -> Minus19/2
  Square8/1 -> Minus19/1
  [D_it] -> Square9/1
  [D_ot] -> Square8/1
  Minus17/1 -> Divide54/1
  Minus18/1 -> Divide52/3
  Constant67/1 -> Divide53/5
  [D_ot] -> Divide53/3
  Constant66/1 -> Divide53/2
  [N] -> Divide53/1
  Divide53/1 -> Divide52/2
  [h_ws] -> Divide52/1
  Divide52/1 -> Minus17/2
  Divide50/1 -> Minus17/1
  Minus16/1 -> Divide50/1
  [h_pw] -> Divide50/2
  Divide51/1 -> Divide50/3
  [N] -> Divide51/1
  Constant64/1 -> Divide51/2
  [D_it] -> Divide51/3
  Constant65/1 -> Divide51/5
  Tp2_otsg/1 -> Minus4/1, [Tp2_otsg], Minus16/1, Minus2/2, Minus3/2
  Tw2_otsg/1 -> Minus16/2, Minus18/2, [Tw2_otsg]
  Tw3_otsg/1 -> [Tw3_otsg], Minus22/2, Minus20/2
  Tp3_otsg/1 -> Minus6/1, [Tp3_otsg], Minus20/1, Minus5/2, Minus4/2
  Constant72/1 -> Divide59/5
  [D_it] -> Divide59/3
  Constant71/1 -> Divide59/2
  [N] -> Divide59/1
  Divide59/1 -> Divide58/3
  [h_pw] -> Divide58/2
  Minus20/1 -> Divide58/1
  Divide58/1 -> Minus21/1
  Divide60/1 -> Minus21/2
  [h_wb] -> Divide60/1
  Divide61/1 -> Divide60/2
  [N] -> Divide61/1
  Constant73/1 -> Divide61/2
  [D_ot] -> Divide61/3
  Constant74/1 -> Divide61/5
  Minus22/1 -> Divide60/3
  Minus21/1 -> Divide62/1
  [D_ot] -> Square10/1
  [D_it] -> Square11/1
  Square10/1 -> Minus23/1
  Square11/1 -> Minus23/2
  Constant76/1 -> Divide64/2
  Minus23/1 -> Divide64/1
  [N] -> Divide63/1
  Constant75/1 -> Divide63/2
  Divide63/1 -> Divide62/2
  Divide64/1 -> Divide63/3
  [rho_w] -> Divide63/4
  [Cp_w] -> Divide63/5
  Divide65/1 -> Divide63/6
  Divide62/1 -> Tw3_otsg/1
  Constant77/1 -> Divide65/2
  Constant84/1 -> Divide73/2
  Divide70/1 -> Tw4_otsg/1
  Divide73/1 -> Divide71/6
  [Cp_w] -> Divide71/5
  [rho_w] -> Divide71/4
  Divide72/1 -> Divide71/3
  Divide71/1 -> Divide70/2
  Constant82/1 -> Divide71/2
  [N] -> Divide71/1
  Minus27/1 -> Divide72/1
  Constant83/1 -> Divide72/2
  Square13/1 -> Minus27/2
  Square12/1 -> Minus27/1
  [D_it] -> Square13/1
  [D_ot] -> Square12/1
  Minus25/1 -> Divide70/1
  Minus26/1 -> Divide68/3
  Constant81/1 -> Divide69/5
  [D_ot] -> Divide69/3
  Constant80/1 -> Divide69/2
  [N] -> Divide69/1
  Divide69/1 -> Divide68/2
  [h_wb] -> Divide68/1
  Divide68/1 -> Minus25/2
  Divide66/1 -> Minus25/1
  Minus24/1 -> Divide66/1
  [h_pw] -> Divide66/2
  Divide67/1 -> Divide66/3
  [N] -> Divide67/1
  Constant78/1 -> Divide67/2
  [D_it] -> Divide67/3
  Constant79/1 -> Divide67/5
  Tp4_otsg/1 -> Minus8/1, Minus24/1, Minus6/2, Minus7/2, [Tp4_otsg]
  Tw4_otsg/1 -> Minus24/2, Minus26/2, [Tw4_otsg]
  Tw5_otsg/1 -> [Tw5_otsg], Minus30/2, Minus28/2
  Tp5_otsg/1 -> Minus10/1, [Tp5_otsg], Minus28/1, Minus9/2, Minus8/2
  Constant86/1 -> Divide75/5
  [D_it] -> Divide75/3
  Constant85/1 -> Divide75/2
  [N] -> Divide75/1
  Divide75/1 -> Divide74/3
  [h_pw] -> Divide74/2
  Minus28/1 -> Divide74/1
  Divide74/1 -> Minus29/1
  Divide76/1 -> Minus29/2
  [h_wsc] -> Divide76/1
  Divide77/1 -> Divide76/2
  [N] -> Divide77/1
  Constant87/1 -> Divide77/2
  [D_ot] -> Divide77/3
  Constant88/1 -> Divide77/5
  Minus30/1 -> Divide76/3
  Minus29/1 -> Divide78/1
  [D_ot] -> Square14/1
  [D_it] -> Square15/1
  Square14/1 -> Minus31/1
  Square15/1 -> Minus31/2
  Constant90/1 -> Divide80/2
  Minus31/1 -> Divide80/1
  [N] -> Divide79/1
  Constant89/1 -> Divide79/2
  Divide79/1 -> Divide78/2
  Divide80/1 -> Divide79/3
  [rho_w] -> Divide79/4
  [Cp_w] -> Divide79/5
  Divide81/1 -> Divide79/6
  Divide78/1 -> Tw5_otsg/1
  Constant91/1 -> Divide81/2
  Constant98/1 -> Divide89/2
  Divide86/1 -> Tw6_otsg/1
  Divide89/1 -> Divide87/6
  [Cp_w] -> Divide87/5
  [rho_w] -> Divide87/4
  Divide88/1 -> Divide87/3
  Divide87/1 -> Divide86/2
  Constant96/1 -> Divide87/2
  [N] -> Divide87/1
  Minus35/1 -> Divide88/1
  Constant97/1 -> Divide88/2
  Square17/1 -> Minus35/2
  Square16/1 -> Minus35/1
  [D_it] -> Square17/1
  [D_ot] -> Square16/1
  Minus33/1 -> Divide86/1
  Minus34/1 -> Divide84/3
  Constant95/1 -> Divide85/5
  [D_ot] -> Divide85/3
  Constant94/1 -> Divide85/2
  [N] -> Divide85/1
  Divide85/1 -> Divide84/2
  [h_wsc] -> Divide84/1
  Divide84/1 -> Minus33/2
  Divide82/1 -> Minus33/1
  Minus32/1 -> Divide82/1
  [h_pw] -> Divide82/2
  Divide83/1 -> Divide82/3
  [N] -> Divide83/1
  Constant92/1 -> Divide83/2
  [D_it] -> Divide83/3
  Constant93/1 -> Divide83/5
  Tp6_otsg/1 -> Minus32/1, Minus10/2, Minus11/2, [Tp6_otsg]
  Tw6_otsg/1 -> Minus32/2, Minus34/2, [Tw6_otsg]
  Divide91/1 -> Product/1
  [Cp_s] -> Product/2
  Constant99/1 -> Divide91/2
  Product/1 -> Divide90/2
  Minus36/1 -> Divide90/1
  Divide92/1 -> Minus36/1
  [h_ws] -> Divide92/3
  Divide93/1 -> Divide92/2
  Constant101/1 -> Divide93/5
  [N] -> Divide93/1
  Constant100/1 -> Divide93/2
  [D_ot] -> Divide93/3
  Minus37/1 -> Divide92/1
  [Tw1_otsg] -> Minus37/1
  Divide94/1 -> Minus36/2
  [Cp_s] -> Divide95/1, Divide94/2
  Minus38/1 -> Divide94/3
  Divide95/1 -> Minus36/3
  Minus39/1 -> Divide95/2
  Constant102/1 -> Divide95/4
  [A_s] -> Divide96/1
  Constant103/1 -> Divide96/3
  Divide96/1 -> Minus40/1
  Constant104/1 -> Divide97/2
  Divide97/1 -> Divide98/1
  [dHs_dPs] -> Divide98/2
  Divide98/1 -> Minus40/2
  Minus40/1 -> Divide99/2
  Divide99/1 -> Minus36/4
  Divide90/1 -> [dTs1_otsg_dt], Ts1_otsg/1
  [Ts1_otsg] -> Steam Temperature/1
  [Tp6_otsg] -> Coolant Salt Outlet Temperature/1
  Divide100/1 -> Ts2_otsg/1, [dTs2_otsg_dt]
  Divide109/1 -> Minus41/3
  Minus45/1 -> Divide109/2
  Divide108/1 -> Minus45/2
  [dHs_dPs] -> Divide108/2
  Divide107/1 -> Divide108/1
  Constant109/1 -> Divide107/2
  Divide106/1 -> Minus45/1
  Constant108/1 -> Divide106/3
  [A_s] -> Divide106/1
  Minus43/1 -> Divide104/3
  [Cp_s] -> Divide104/2
  Divide104/1 -> Minus41/2
  [Tw2_otsg] -> Minus42/1
  Minus42/1 -> Divide102/1
  [D_ot] -> Divide103/3
  Constant105/1 -> Divide103/2
  [N] -> Divide103/1
  Constant106/1 -> Divide103/5
  Divide103/1 -> Divide102/2
  [h_ws] -> Divide102/3
  Divide102/1 -> Minus41/1
  Minus41/1 -> Divide100/1
  Product1/1 -> Divide100/2
  Constant110/1 -> Divide101/2
  [Cp_s] -> Product1/2
  Divide101/1 -> Product1/1
  Ts2_otsg/1 -> Minus39/1, Minus38/1, Minus42/2, Minus43/2, [Ts2_otsg]
  Divide105/1 -> Tsc2_otsg/1
  [L_sc] -> Divide105/2
  Minus44/1 -> Divide105/1
  Divide110/1 -> Minus44/1
  Product2/1 -> Divide110/3
  Constant107/1 -> Divide110/1
  Product3/1 -> Minus44/2
  [A_s] -> Product2/1
  [rho_sc] -> Product2/2
  [Cp_sc] -> Product2/3
  Minus46/1 -> Divide110/2
  [h_wsc] -> Divide111/1
  [N] -> Divide111/2
  Constant111/1 -> Divide111/3
  [D_ot] -> Divide111/4
  Constant112/1 -> Divide111/7
  Minus47/1 -> Divide111/6
  [Tw6_otsg] -> Minus47/1
  Divide111/1 -> Minus46/1
  [A_s] -> Divide112/1
  Constant113/1 -> Divide112/4
  Divide112/1 -> Minus46/3
  [Cp_sc] -> Divide113/1
  Minus48/1 -> Divide113/2
  Divide114/1 -> Minus48/1
  Divide115/1 -> Minus48/2
  [Wfw_in] -> Divide114/1
  [Tfw_in] -> Divide114/2
  Constant114/1 -> Divide115/2
  Minus49/1 -> Divide115/1
  [Wfw_in] -> Minus49/1
  Divide113/1 -> Minus46/2
  Constant115/1 -> Plus6/1
  Multiply/1 -> Plus6/2
  Plus6/1 -> Unit Delay/1  "rho_b(Ps)"
  Minus50/1 -> Unit Delay1/1  "Steam Level"
  [L] -> Minus50/1
  Divide116/1 -> Minus51/1
  Constant116/1 -> Divide116/1
  Minus51/1 -> [dL_s_dt]  "dLs/dt"
  Product4/1 -> Divide117/2
  [A_s] -> Product4/1
  Minus52/1 -> Divide117/1
  [A_s] -> Product5/1
  Product5/1 -> Minus52/3
  [K_b] -> Product5/3
  Divide117/1 -> [dL_b_dt], L_b/1  "dLb/dt"
  Constant117/1 -> Divide118/1
  [A_s] -> Divide119/1
  Constant118/1 -> Divide119/2
  [rho_sc] -> Divide119/3
  [Cp_sc] -> Divide119/4
  [Tsc2_otsg] -> Minus53/1
  Minus53/1 -> Divide119/5
  Divide119/1 -> Divide118/2
  Divide118/1 -> Divide120/1
  Minus54/1 -> Divide120/2
  [Wfw_in] -> Minus56/1
  Minus56/1 -> Divide123/1
  Constant119/1 -> Divide123/2
  [Tsc2_otsg] -> Divide122/2
  [Wfw_in] -> Divide122/1
  Divide123/1 -> Minus55/2
  Divide122/1 -> Minus55/1
  Minus55/1 -> Divide121/2
  [Cp_sc] -> Divide121/1
  Divide124/1 -> Minus54/1
  [h_wsc] -> Divide124/1
  [N] -> Divide124/2
  Constant120/1 -> Divide124/3
  [D_ot] -> Divide124/4
  Constant121/1 -> Divide124/7
  Minus57/1 -> Divide124/6
  [Tw5_otsg] -> Minus57/1
  Divide121/1 -> Minus54/2
  [A_s] -> Divide125/1
  Constant122/1 -> Divide125/5
  Minus58/1 -> Divide125/3
  Constant123/1 -> Minus58/2
  Divide126/1 -> Minus58/1
  [K_sc] -> Divide126/1
  [Cp_sc] -> Divide126/2
  Minus59/1 -> Divide126/3
  [Tsc2_otsg] -> Minus59/1
  Divide127/1 -> Minus59/2
  Constant124/1 -> Divide127/1
  Divide125/1 -> Minus54/3
  Divide128/1 -> Minus54/4
  [A_s] -> Divide128/1
  [rho_sc] -> Divide128/2
  [Cp_sc] -> Divide128/3
  [K_1] -> Divide128/4
  Constant125/1 -> Divide128/7
  Divide120/1 -> L_sc/1, [dL_sc_dt]  "dLsc/dt"
  Divide129/1 -> [dP_s_dt], P_s/1  "dPs/dt"
  Divide130/1 -> Divide129/2
  [A_s] -> Divide130/1
  [L_s] -> Divide130/2
  Minus60/1 -> Divide129/1
  P_s/1 -> Divide131/1, [P_s]  "Ps = Steam Pressure"
  Divide131/1 -> Minus60/2
  [A_s] -> Divide131/2
  [dL_s_dt] -> Divide131/3
  Divide132/1 -> Minus60/1
  Constant126/1 -> Divide132/5
  [M_stm] -> Divide132/4
  [Z_ss] -> Divide132/3
  [R] -> Divide132/2
  Product7/1 -> Minus61/2
  Product6/1 -> Minus61/1
  Minus61/1 -> Divide132/1
  Sum/1 -> Product6/2
  [Ts1_otsg] -> Sum/2
  [Ts2_otsg] -> Sum/1
  Sum1/1 -> Product7/1
  [dTs2_otsg_dt] -> Sum1/2
  [dTs1_otsg_dt] -> Sum1/1
  [P_s] -> Steam Pressure/1
  [dP_s_dt] -> P_sat/1, [dP_sat_dt]  "dPsat/dt"
  [dP_s_dt] -> [dP_sc_dt], P_sc/1  "dPsc/dt"
  P_sc/1 -> [P_sc]  "Subcooled Pressure"
  [K_5] -> Product8/1
  [P_sat] -> Product8/2
  Minus62/1 -> [T_sat]  "Tsat"
  [X_5] -> Minus62/1
  Product8/1 -> Minus62/2
  Minus63/1 -> M_shs/1, [dM_shs_dt]  "rate of change of superheated steam mass"
  Divide133/1 -> Unit Delay2/1
  [Wfw_in] -> Divide133/1
  [P_set_point] -> Divide133/3
  [P_s] -> Divide133/2
  Minus64/1 -> [W_db]  "flow rate from subcooled to boiling region"
  [Wfw_in] -> Minus64/1
  [rho_sc] -> Divide134/1
  [A_s] -> Divide134/2
  Divide134/1 -> Minus64/2
  [dL_sc_dt] -> Divide134/3
  [A_s] -> Divide135/1
  [L_sc] -> Divide135/2
  [K_sc] -> Divide135/3
  [dP_sc_dt] -> Divide135/4
  Divide135/1 -> Minus64/3
  Divide136/1 -> [W_b]  "flow rate from boiling to superheating region"
  [K_4] -> Product9/1
  [P_sat] -> Product9/2
  Product9/1 -> Minus65/2
  [X_4] -> Minus65/1
  Minus65/1 -> Divide136/2
  Divide137/1 -> Divide136/1
  [h_wb] -> Divide137/6
  [N] -> Divide137/5
  [D_ot] -> Divide137/4
  Constant127/1 -> Divide137/3
  [L_b] -> Divide137/2
  Minus66/1 -> Divide137/1
  [T_sat] -> Minus66/3
  Product10/1 -> Minus66/2
  Constant129/1 -> Product10/1
  [Tw4_otsg] -> Product10/2
  Constant128/1 -> Product11/1
  [Tw3_otsg] -> Product11/2
  Product11/1 -> Minus66/1
  [L_s] -> Divide4/4
  [Tw1_otsg] -> Minus1/1
  [L_s] -> Divide6/1
  [L_s] -> Divide11/4
  [Tw2_otsg] -> Minus3/1
  [L_s] -> Divide13/1
  [L_b] -> Divide15/4
  [L_b] -> Divide17/1
  [Tw3_otsg] -> Minus5/1
  [L_b] -> Divide22/4
  [L_b] -> Divide24/1
  [Tw4_otsg] -> Minus7/1
  [L_sc] -> Divide29/4
  [L_sc] -> Divide31/1
  [Tw5_otsg] -> Minus9/1
  [Tw6_otsg] -> Minus11/1
  [L_sc] -> Divide36/4
  [L_sc] -> Divide38/1
  [L_s] -> Divide43/4
  [L_s] -> Divide45/4
  [L_s] -> Divide49/1
  [L_s] -> Divide51/4
  [L_s] -> Divide53/4
  [L_s] -> Divide57/1
  [Ts1_otsg] -> Minus14/1
  [Ts2_otsg] -> Minus18/1
  [L_b] -> Divide59/4
  [L_b] -> Divide65/1
  [L_b] -> Divide61/4
  [T_sat] -> Minus22/1
  [T_sat] -> Minus26/1
  [L_b] -> Divide73/1
  [L_b] -> Divide69/4
  [L_b] -> Divide67/4
  [L_sc] -> Divide75/4
  [L_sc] -> Divide77/4
  [L_sc] -> Divide81/1
  [T_sat] -> Minus30/1
  [L_sc] -> Divide83/4
  [L_sc] -> Divide85/4
  [L_sc] -> Divide89/1
  [Tsc2_otsg] -> Minus34/1
  [L_s] -> Divide93/4
  [M_s_fac1] -> Divide94/1
  [dM_shs_dt] -> Divide95/3
  [L_s] -> Divide96/2
  [M_shs] -> Divide97/1
  [dP_s_dt] -> Divide99/1
  [M_shs] -> Divide91/1
  [L_s] -> Divide103/4
  [W_b] -> Divide104/1
  [T_sat] -> Minus43/1
  [L_s] -> Divide106/2
  [M_shs] -> Divide107/1
  [dP_s_dt] -> Divide109/1
  [M_shs] -> Divide101/1
  [L_sc] -> Divide111/5
  [L_sc] -> Divide112/2
  [dP_sc_dt] -> Divide112/3
  [W_db] -> Minus49/2
  [dL_sc_dt] -> Product3/2
  [P_s] -> Multiply/1
  [L_b] -> Minus50/2
  [L_sc] -> Minus50/3
  [dL_b_dt] -> Divide116/2
  [dL_sc_dt] -> Minus51/2
  [W_db] -> Minus52/1
  [W_b] -> Minus52/2
  [L_b] -> Product5/2
  [dP_sat_dt] -> Product5/4
  [T_sat] -> Minus53/2
  [T_sat] -> Minus57/2
  [L_sc] -> Divide124/5
  [W_db] -> Minus56/2
  [L_sc] -> Divide125/2
  [T_sat] -> Divide123/3
  [T_sat] -> Divide127/2
  [dP_sc_dt] -> Divide125/4
  [L_sc] -> Divide128/5
  [dP_sat_dt] -> Divide128/6
  [dM_shs_dt] -> Product6/1
  [M_shs] -> Product7/2
  [W_b] -> Minus63/1
  [M_s_fac1] -> Minus63/2
  Unit Delay2/1 -> [Steam_flow_rate], [M_s_fac1]
  [Steam_flow_rate] -> Steam Flow Rate/1
  Mux/1 -> Unit Delay3/1
  Unit Delay3/1 -> To Workspace/1
  [Tp_in] -> Mux1/1, OTSG Primary Temps/1, Mux/1
  [Tfw_in] -> Mux3/1, Feedwater and steam Temps/1, Mux/2
  [Wp_in] -> Mux/3
  [cool_hA_frac] -> Mux/4
  [P_set_point] -> Mux/6
  [Tp1_otsg] -> Mux1/2, OTSG Primary Temps/2, Mux/7
  [Tp2_otsg] -> Mux1/3, OTSG Primary Temps/3, Mux/8
  [Tp3_otsg] -> Mux1/4, OTSG Primary Temps/4, Mux/9
  [Tp4_otsg] -> Mux1/5, OTSG Primary Temps/5, Mux/10
  [Tp5_otsg] -> Mux1/6, OTSG Primary Temps/6, Mux/11
  [Tp6_otsg] -> Mux1/7, OTSG Primary Temps/7, Mux/12
  [Tw1_otsg] -> Mux2/1, OTSG Tube Temps/1, Mux/13
  [Tw2_otsg] -> Mux2/2, OTSG Tube Temps/2, Mux/14
  [Tw3_otsg] -> Mux2/3, OTSG Tube Temps/3, Mux/15
  [Tw4_otsg] -> Mux2/4, OTSG Tube Temps/4, Mux/16
  [Tw5_otsg] -> Mux2/5, OTSG Tube Temps/5, Mux/17
  [Tw6_otsg] -> Mux2/6, OTSG Tube Temps/6, Mux/18
  [Ts1_otsg] -> Feedwater and steam Temps/4, Mux3/4, Mux/19
  [dTs1_otsg_dt] -> Mux/20
  [Ts2_otsg] -> Mux3/5, Feedwater and steam Temps/3, Mux/21
  [dTs2_otsg_dt] -> Mux/22
  [Tsc2_otsg] -> Feedwater and steam Temps/2, Mux3/2, Mux/23
  [L_b] -> Mux4/2, OTSG Level/2, Mux/28
  [dL_b_dt] -> Mux/27
  [rho_b_Ps] -> Mux/24, To Workspace4/1, Density of Boiling/1
  [dL_s_dt] -> Mux/26
  [L_s] -> Mux4/1, OTSG Level/1, Mux/25
  [dL_sc_dt] -> Mux/29
  [L_sc] -> Mux4/3, OTSG Level/3, Mux/30
  [dP_s_dt] -> Mux/31
  [P_s] -> Mux5/1, Feedwater and Steam Pressures/1, Mux/32
  [dP_sat_dt] -> Mux/33
  [P_sat] -> Mux5/2, Feedwater and Steam Pressures/2, Mux/34
  [dP_sc_dt] -> Mux/35
  [P_sc] -> Mux5/3, Feedwater and Steam Pressures/3, Mux/36
  [dM_shs_dt] -> Mux/38
  [M_shs] -> Mux/39
  [M_s_fac1] -> Feedwater and Steam Flow Rates/4, Mux6/4, Mux/40
  [W_db] -> Feedwater and Steam Flow Rates/2, Mux6/2, Mux/41
  [cool_hA_frac] -> Divide1/4
  [cool_hA_frac] -> Divide42/4
  [cool_hA_frac] -> Divide8/4
  [cool_hA_frac] -> Divide50/4
  [cool_hA_frac] -> Divide19/4
  [cool_hA_frac] -> Divide58/4
  [cool_hA_frac] -> Divide26/4
  [cool_hA_frac] -> Divide66/4
  [cool_hA_frac] -> Divide33/4
  [cool_hA_frac] -> Divide74/4
  [cool_hA_frac] -> Divide40/4
  [cool_hA_frac] -> Divide82/4
  [T_sat] -> Feedwater and steam Temps/5, Mux3/3, Mux/37
  Mux1/1 -> To Workspace1/1
  Mux2/1 -> To Workspace2/1
  Mux3/1 -> To Workspace3/1
  Mux4/1 -> To Workspace5/1
  Mux5/1 -> To Workspace6/1
  [Wfw_in] -> Mux/5, Mux6/1, Feedwater and Steam Flow Rates/1
  [W_b] -> Feedwater and Steam Flow Rates/3, Mux6/3, Mux/42
  Mux6/1 -> To Workspace7/1
